simulink model "HVDC_VSC_1CPUcore_dcpl"  (Simulink 8.4)
settings: Solver=ode3  SolverMode=SingleTasking  StartTime=0.0  StopTime=70.0  FixedStep=Ts_Power  RelTol=1e-3  AbsTol=1e-2
PreLoadFcn:
  | Ts_Power=50e-6; Ts_Control=1*Ts_Power; init_cosim_IA; startup_transients_hvdc_vsc;
PostLoadFcn:
  | Ts_Power=50e-6; Ts_Control=1*Ts_Power; init_cosim_IA; startup_transients_hvdc_vsc;
InitFcn:
  | Ts_Power=50e-6; Ts_Control=1*Ts_Power; init_cosim_IA; startup_transients_hvdc_vsc;
undefined symbols (not defined in the file): CLARK, D1, Delta, dPref1_2, dPref1_2_rlimit, gcbh, h, intfDelay, level, lib_mesures, magnitude, ResistanceM, rte_drive_private_lib, rte_tsb3level_hiz_rect_cb, sps_rtmsupport, t_deblock_Pref1, t_deblock_Udref2, t_dPref1_2, t_SwitchITMIdc, t_SwitchITMVdc, Ts_intf, TSB3_hiZR
libraries: powerlib x183, spsVIMeasurementModel x102, powerlib_extras x71, powerlib_meascontrol x50, rteventslib x26, op_dpl_lib x20, rtlab x14, sps_avr x6, artemis x1
(part 8 of 13)

== system HVDC_VSC_1CPUcore_dcpl/SS_HVDCStation2_WSCC2/WSCC System 2/Bus_4 230 KV ==
  Three-Phase V-I Measurement1 : Subsystem  DialogController=POWERSYS.PowerSysDialog  LoadFcn=sps_rtmsupport('LoadFcn',gcbh);  StartFcn=sps_rtmsupport('StartFcn',gcbh);  StopFcn=sps_rtmsupport('StopFcn',gcbh);  mask(Three-Phase VI Measurement){VoltageMeasurement=phase-to-phase, SetLabelV=on, LabelV=Vabc_245, Vpu=off, VpuLL=off, CurrentMeasurement=yes, SetLabelI=on, LabelI=Iabc_245, Ipu=off, Pbase=100e6, Vbase=230e3, OutputType=Complex, PhasorSimulation=off, PSBequivalent=0}
      mask prompts: VoltageMeasurement "Voltage measurement"; SetLabelV "Use a label"; LabelV "Signal label  (use a From block to collect this signal)"; Vpu "Voltages in pu,  based on peak value of nominal phase-to-ground voltage"; VpuLL "Voltages in pu,  based on peak value of nominal phase-to-phase  voltage"; CurrentMeasurement "Current measurement"; SetLabelI "Use a label"; LabelI "Signal label  (use a From block to collect this signal)"; Ipu "Currents in pu"; Pbase "Base power ( VA 3 phase)"; Vbase "Nominal voltage used for pu measurement (Vrms phase-phase) :"; OutputType "Output signals in:"; PhasorSimulation "Phasor simulation (internal use)"; PSBequivalent "Equivalent circuit (internal use)"
      mask help:
      | Ideal three-phase voltage and current measurements.
      |
      | The block can output the voltages and currents in per unit values or in volts and amperes.
      mask init: same as HVDC_VSC_1CPUcore_dcpl/SM_WSCC1_HVDCStation1/B1
      settings: CopyFcn=sps_rtmsupport('CopyFcn',gcbh); powericon('ThreePhaseVIMeasurementCopy',gcb)  DeleteFcn=sps_rtmsupport('DeleteFcn',gcbh);  UndoDeleteFcn=sps_rtmsupport('UndoDeleteFcn',gcbh);  ModelCloseFcn=sps_rtmsupport('ModelCloseFcn',gcbh);  PreSaveFcn="sps_rtmsupport('PreSaveFcn',gcbh);  set_param(gcb,'LinkStatus','restore')"  PostSaveFcn=sps_rtmsupport('PostSaveFcn',gcbh);  NameChangeFcn=sps_rtmsupport('NameChangeFcn',gcbh);  PreCopyFcn=sps_rtmsupport('PreCopyFcn',gcbh);  OpenFcn=sps_rtmsupport('OpenFcn',gcbh, [1 2 4 5 6 7 9 -12 13]);  CloseFcn=sps_rtmsupport('CloseFcn',gcbh);  PreDeleteFcn=sps_rtmsupport('PreDeleteFcn',gcbh);
      mask Help: helpview(psbhelp)
      mask TypeOptions VoltageMeasurement: no | phase-to-ground | phase-to-phase
      mask Callback VoltageMeasurement: powericon('ThreePhaseVIMeasurementCback',gcb,'Vselector');
      mask Callback SetLabelV: powericon('ThreePhaseVIMeasurementCback',gcb,'');
      mask Callback Vpu: powericon('ThreePhaseVIMeasurementCback',gcb,'Vpu');
      mask Callback VpuLL: powericon('ThreePhaseVIMeasurementCback',gcb,'VpuLL');
      mask TypeOptions CurrentMeasurement: no | yes
      mask Callback CurrentMeasurement: powericon('ThreePhaseVIMeasurementCback',gcb,'');
      mask Callback SetLabelI: powericon('ThreePhaseVIMeasurementCback',gcb,'');
      mask Callback LabelI: powericon('ThreePhaseVIMeasurementCback',gcb,'');
      mask Callback Ipu: powericon('ThreePhaseVIMeasurementCback',gcb,'');
      mask TypeOptions OutputType: Complex | Real-Imag | Magnitude-Angle | Magnitude
  Three-Phase V-I Measurement3 : Subsystem  DialogController=POWERSYS.PowerSysDialog  LoadFcn=sps_rtmsupport('LoadFcn',gcbh);  StartFcn=sps_rtmsupport('StartFcn',gcbh);  StopFcn=sps_rtmsupport('StopFcn',gcbh);  mask(Three-Phase VI Measurement){VoltageMeasurement=phase-to-phase, SetLabelV=on, LabelV=Vabc_246, Vpu=off, VpuLL=off, CurrentMeasurement=yes, SetLabelI=on, LabelI=Iabc_246, Ipu=off, Pbase=100e6, Vbase=230e3, OutputType=Complex, PhasorSimulation=off, PSBequivalent=0}
      mask prompts: VoltageMeasurement "Voltage measurement"; SetLabelV "Use a label"; LabelV "Signal label  (use a From block to collect this signal)"; Vpu "Voltages in pu,  based on peak value of nominal phase-to-ground voltage"; VpuLL "Voltages in pu,  based on peak value of nominal phase-to-phase  voltage"; CurrentMeasurement "Current measurement"; SetLabelI "Use a label"; LabelI "Signal label  (use a From block to collect this signal)"; Ipu "Currents in pu"; Pbase "Base power ( VA 3 phase)"; Vbase "Nominal voltage used for pu measurement (Vrms phase-phase) :"; OutputType "Output signals in:"; PhasorSimulation "Phasor simulation (internal use)"; PSBequivalent "Equivalent circuit (internal use)"
      mask help:
      | Ideal three-phase voltage and current measurements.
      |
      | The block can output the voltages and currents in per unit values or in volts and amperes.
      mask init: same as HVDC_VSC_1CPUcore_dcpl/SM_WSCC1_HVDCStation1/B1
      settings: CopyFcn=sps_rtmsupport('CopyFcn',gcbh); powericon('ThreePhaseVIMeasurementCopy',gcb)  DeleteFcn=sps_rtmsupport('DeleteFcn',gcbh);  UndoDeleteFcn=sps_rtmsupport('UndoDeleteFcn',gcbh);  ModelCloseFcn=sps_rtmsupport('ModelCloseFcn',gcbh);  PreSaveFcn="sps_rtmsupport('PreSaveFcn',gcbh);  set_param(gcb,'LinkStatus','restore')"  PostSaveFcn=sps_rtmsupport('PostSaveFcn',gcbh);  NameChangeFcn=sps_rtmsupport('NameChangeFcn',gcbh);  PreCopyFcn=sps_rtmsupport('PreCopyFcn',gcbh);  OpenFcn=sps_rtmsupport('OpenFcn',gcbh, [1 2 4 5 6 7 9 -12 13]);  CloseFcn=sps_rtmsupport('CloseFcn',gcbh);  PreDeleteFcn=sps_rtmsupport('PreDeleteFcn',gcbh);
      mask Help: helpview(psbhelp)
      mask TypeOptions VoltageMeasurement: no | phase-to-ground | phase-to-phase
      mask Callback VoltageMeasurement: powericon('ThreePhaseVIMeasurementCback',gcb,'Vselector');
      mask Callback SetLabelV: powericon('ThreePhaseVIMeasurementCback',gcb,'');
      mask Callback Vpu: powericon('ThreePhaseVIMeasurementCback',gcb,'Vpu');
      mask Callback VpuLL: powericon('ThreePhaseVIMeasurementCback',gcb,'VpuLL');
      mask TypeOptions CurrentMeasurement: no | yes
      mask Callback CurrentMeasurement: powericon('ThreePhaseVIMeasurementCback',gcb,'');
      mask Callback SetLabelI: powericon('ThreePhaseVIMeasurementCback',gcb,'');
      mask Callback LabelI: powericon('ThreePhaseVIMeasurementCback',gcb,'');
      mask Callback Ipu: powericon('ThreePhaseVIMeasurementCback',gcb,'');
      mask TypeOptions OutputType: Complex | Real-Imag | Magnitude-Angle | Magnitude
  Conn7 : PMIOPort  Port=1  Side=Left
  Conn8 : PMIOPort  Port=2  Side=Left
  Conn9 : PMIOPort  Port=3  Side=Left
  Conn1 : PMIOPort  Port=4  Side=Right
  Conn2 : PMIOPort  Port=5  Side=Right
  Conn3 : PMIOPort  Port=6  Side=Right
  Conn4 : PMIOPort  Port=7  Side=Right
  Conn5 : PMIOPort  Port=8  Side=Right
  Conn6 : PMIOPort  Port=9  Side=Right
  connections:
  Three-Phase V-I Measurement3/LConn3 -- Conn9/RConn1 -- Three-Phase V-I Measurement1/LConn3
  Three-Phase V-I Measurement3/LConn2 -- Conn8/RConn1 -- Three-Phase V-I Measurement1/LConn2
  Three-Phase V-I Measurement3/LConn1 -- Conn7/RConn1 -- Three-Phase V-I Measurement1/LConn1
  Three-Phase V-I Measurement3/RConn3 -- Conn6/RConn1
  Three-Phase V-I Measurement1/RConn3 -- Conn3/RConn1
  Three-Phase V-I Measurement1/RConn1 -- Conn1/RConn1
  Three-Phase V-I Measurement1/RConn2 -- Conn2/RConn1
  Three-Phase V-I Measurement3/RConn1 -- Conn4/RConn1
  Three-Phase V-I Measurement3/RConn2 -- Conn5/RConn1

== system HVDC_VSC_1CPUcore_dcpl/SS_HVDCStation2_WSCC2/WSCC System 2/Bus_5 230 KV ==
  Kv : Gain  Gain=Ki  SaturateOnIntegerOverflow=on  OutDataTypeStr=Inherit: Same as input  ParamDataTypeStr=Inherit: Same as input
  Kv1 : Gain  Gain=Kv  SaturateOnIntegerOverflow=on  OutDataTypeStr=Inherit: Same as input  ParamDataTypeStr=Inherit: Same as input
  Mode I : spsVIMeasurementModel/Complex
  Mode V : spsVIMeasurementModel/Complex
  Model : spsVIMeasurementModel/VI_phase  SystemSampleTime=-1
  A : PMIOPort  Port=1  Side=Left
  B : PMIOPort  Port=2  Side=Left
  C : PMIOPort  Port=3  Side=Left
  a : PMIOPort  Port=4  Side=Right
  b : PMIOPort  Port=5  Side=Right
  c : PMIOPort  Port=6  Side=Right
  tag scope: Iabc_25=global, Vabc_25=global
  wires:
  Model/2 -> Kv/1
  Model/1 -> Kv1/1
  Kv/1 -> Mode I/1
  Kv1/1 -> Mode V/1
  Mode I/1 -> [Iabc_25]
  Mode V/1 -> [Vabc_25]
  connections:
  Model/RConn3 -- c/RConn1
  Model/RConn1 -- a/RConn1
  Model/RConn2 -- b/RConn1
  Model/LConn3 -- C/RConn1
  Model/LConn1 -- A/RConn1
  Model/LConn2 -- B/RConn1

== system HVDC_VSC_1CPUcore_dcpl/SS_HVDCStation2_WSCC2/WSCC System 2/Bus_6 230 KV ==
  Kv : Gain  Gain=Ki  SaturateOnIntegerOverflow=on  OutDataTypeStr=Inherit: Same as input  ParamDataTypeStr=Inherit: Same as input
  Kv1 : Gain  Gain=Kv  SaturateOnIntegerOverflow=on  OutDataTypeStr=Inherit: Same as input  ParamDataTypeStr=Inherit: Same as input
  Mode I : spsVIMeasurementModel/Complex
  Mode V : spsVIMeasurementModel/Complex
  Model : spsVIMeasurementModel/VI_phase  SystemSampleTime=-1
  A : PMIOPort  Port=1  Side=Left
  B : PMIOPort  Port=2  Side=Left
  C : PMIOPort  Port=3  Side=Left
  a : PMIOPort  Port=4  Side=Right
  b : PMIOPort  Port=5  Side=Right
  c : PMIOPort  Port=6  Side=Right
  tag scope: Iabc_26=global, Vabc_26=global
  wires:
  Model/2 -> Kv/1
  Model/1 -> Kv1/1
  Kv/1 -> Mode I/1
  Kv1/1 -> Mode V/1
  Mode I/1 -> [Iabc_26]
  Mode V/1 -> [Vabc_26]
  connections:
  Model/RConn3 -- c/RConn1
  Model/RConn1 -- a/RConn1
  Model/RConn2 -- b/RConn1
  Model/LConn3 -- C/RConn1
  Model/LConn1 -- A/RConn1
  Model/LConn2 -- B/RConn1

== system HVDC_VSC_1CPUcore_dcpl/SS_HVDCStation2_WSCC2/WSCC System 2/Bus_7 230 KV ==
  Three-Phase V-I Measurement1 : Subsystem  DialogController=POWERSYS.PowerSysDialog  LoadFcn=sps_rtmsupport('LoadFcn',gcbh);  StartFcn=sps_rtmsupport('StartFcn',gcbh);  StopFcn=sps_rtmsupport('StopFcn',gcbh);  mask(Three-Phase VI Measurement){VoltageMeasurement=phase-to-phase, SetLabelV=on, LabelV=Vabc_27, Vpu=off, VpuLL=off, CurrentMeasurement=yes, SetLabelI=on, LabelI=Iabc_27, Ipu=off, Pbase=100e6, Vbase=230e3, OutputType=Complex, PhasorSimulation=off, PSBequivalent=0}
      mask prompts: VoltageMeasurement "Voltage measurement"; SetLabelV "Use a label"; LabelV "Signal label  (use a From block to collect this signal)"; Vpu "Voltages in pu,  based on peak value of nominal phase-to-ground voltage"; VpuLL "Voltages in pu,  based on peak value of nominal phase-to-phase  voltage"; CurrentMeasurement "Current measurement"; SetLabelI "Use a label"; LabelI "Signal label  (use a From block to collect this signal)"; Ipu "Currents in pu"; Pbase "Base power ( VA 3 phase)"; Vbase "Nominal voltage used for pu measurement (Vrms phase-phase) :"; OutputType "Output signals in:"; PhasorSimulation "Phasor simulation (internal use)"; PSBequivalent "Equivalent circuit (internal use)"
      mask help:
      | Ideal three-phase voltage and current measurements.
      |
      | The block can output the voltages and currents in per unit values or in volts and amperes.
      mask init: same as HVDC_VSC_1CPUcore_dcpl/SM_WSCC1_HVDCStation1/B1
      settings: CopyFcn=sps_rtmsupport('CopyFcn',gcbh); powericon('ThreePhaseVIMeasurementCopy',gcb)  DeleteFcn=sps_rtmsupport('DeleteFcn',gcbh);  UndoDeleteFcn=sps_rtmsupport('UndoDeleteFcn',gcbh);  ModelCloseFcn=sps_rtmsupport('ModelCloseFcn',gcbh);  PreSaveFcn="sps_rtmsupport('PreSaveFcn',gcbh);  set_param(gcb,'LinkStatus','restore')"  PostSaveFcn=sps_rtmsupport('PostSaveFcn',gcbh);  NameChangeFcn=sps_rtmsupport('NameChangeFcn',gcbh);  PreCopyFcn=sps_rtmsupport('PreCopyFcn',gcbh);  OpenFcn=sps_rtmsupport('OpenFcn',gcbh, [1 2 4 5 6 7 9 -12 13]);  CloseFcn=sps_rtmsupport('CloseFcn',gcbh);  PreDeleteFcn=sps_rtmsupport('PreDeleteFcn',gcbh);
      mask Help: helpview(psbhelp)
      mask TypeOptions VoltageMeasurement: no | phase-to-ground | phase-to-phase
      mask Callback VoltageMeasurement: powericon('ThreePhaseVIMeasurementCback',gcb,'Vselector');
      mask Callback SetLabelV: powericon('ThreePhaseVIMeasurementCback',gcb,'');
      mask Callback Vpu: powericon('ThreePhaseVIMeasurementCback',gcb,'Vpu');
      mask Callback VpuLL: powericon('ThreePhaseVIMeasurementCback',gcb,'VpuLL');
      mask TypeOptions CurrentMeasurement: no | yes
      mask Callback CurrentMeasurement: powericon('ThreePhaseVIMeasurementCback',gcb,'');
      mask Callback SetLabelI: powericon('ThreePhaseVIMeasurementCback',gcb,'');
      mask Callback LabelI: powericon('ThreePhaseVIMeasurementCback',gcb,'');
      mask Callback Ipu: powericon('ThreePhaseVIMeasurementCback',gcb,'');
      mask TypeOptions OutputType: Complex | Real-Imag | Magnitude-Angle | Magnitude
  Three-Phase V-I Measurement3 : Subsystem  DialogController=POWERSYS.PowerSysDialog  LoadFcn=sps_rtmsupport('LoadFcn',gcbh);  StartFcn=sps_rtmsupport('StartFcn',gcbh);  StopFcn=sps_rtmsupport('StopFcn',gcbh);  mask(Three-Phase VI Measurement){VoltageMeasurement=phase-to-phase, SetLabelV=on, LabelV=Vabc_20, Vpu=off, VpuLL=off, CurrentMeasurement=yes, SetLabelI=on, LabelI=Iab_20, Ipu=off, Pbase=100e6, Vbase=230e3, OutputType=Complex, PhasorSimulation=off, PSBequivalent=0}
      mask prompts: VoltageMeasurement "Voltage measurement"; SetLabelV "Use a label"; LabelV "Signal label  (use a From block to collect this signal)"; Vpu "Voltages in pu,  based on peak value of nominal phase-to-ground voltage"; VpuLL "Voltages in pu,  based on peak value of nominal phase-to-phase  voltage"; CurrentMeasurement "Current measurement"; SetLabelI "Use a label"; LabelI "Signal label  (use a From block to collect this signal)"; Ipu "Currents in pu"; Pbase "Base power ( VA 3 phase)"; Vbase "Nominal voltage used for pu measurement (Vrms phase-phase) :"; OutputType "Output signals in:"; PhasorSimulation "Phasor simulation (internal use)"; PSBequivalent "Equivalent circuit (internal use)"
      mask help:
      | Ideal three-phase voltage and current measurements.
      |
      | The block can output the voltages and currents in per unit values or in volts and amperes.
      mask init: same as HVDC_VSC_1CPUcore_dcpl/SM_WSCC1_HVDCStation1/B1
      settings: CopyFcn=sps_rtmsupport('CopyFcn',gcbh); powericon('ThreePhaseVIMeasurementCopy',gcb)  DeleteFcn=sps_rtmsupport('DeleteFcn',gcbh);  UndoDeleteFcn=sps_rtmsupport('UndoDeleteFcn',gcbh);  ModelCloseFcn=sps_rtmsupport('ModelCloseFcn',gcbh);  PreSaveFcn="sps_rtmsupport('PreSaveFcn',gcbh);  set_param(gcb,'LinkStatus','restore')"  PostSaveFcn=sps_rtmsupport('PostSaveFcn',gcbh);  NameChangeFcn=sps_rtmsupport('NameChangeFcn',gcbh);  PreCopyFcn=sps_rtmsupport('PreCopyFcn',gcbh);  OpenFcn=sps_rtmsupport('OpenFcn',gcbh, [1 2 4 5 6 7 9 -12 13]);  CloseFcn=sps_rtmsupport('CloseFcn',gcbh);  PreDeleteFcn=sps_rtmsupport('PreDeleteFcn',gcbh);
      mask Help: helpview(psbhelp)
      mask TypeOptions VoltageMeasurement: no | phase-to-ground | phase-to-phase
      mask Callback VoltageMeasurement: powericon('ThreePhaseVIMeasurementCback',gcb,'Vselector');
      mask Callback SetLabelV: powericon('ThreePhaseVIMeasurementCback',gcb,'');
      mask Callback Vpu: powericon('ThreePhaseVIMeasurementCback',gcb,'Vpu');
      mask Callback VpuLL: powericon('ThreePhaseVIMeasurementCback',gcb,'VpuLL');
      mask TypeOptions CurrentMeasurement: no | yes
      mask Callback CurrentMeasurement: powericon('ThreePhaseVIMeasurementCback',gcb,'');
      mask Callback SetLabelI: powericon('ThreePhaseVIMeasurementCback',gcb,'');
      mask Callback LabelI: powericon('ThreePhaseVIMeasurementCback',gcb,'');
      mask Callback Ipu: powericon('ThreePhaseVIMeasurementCback',gcb,'');
      mask TypeOptions OutputType: Complex | Real-Imag | Magnitude-Angle | Magnitude
  Conn7 : PMIOPort  Port=1  Side=Left
  Conn8 : PMIOPort  Port=2  Side=Left
  Conn9 : PMIOPort  Port=3  Side=Left
  Conn1 : PMIOPort  Port=4  Side=Right
  Conn2 : PMIOPort  Port=5  Side=Right
  Conn3 : PMIOPort  Port=6  Side=Right
  Conn4 : PMIOPort  Port=7  Side=Right
  Conn5 : PMIOPort  Port=8  Side=Right
  Conn6 : PMIOPort  Port=9  Side=Right
  connections:
  Three-Phase V-I Measurement3/RConn2 -- Conn5/RConn1
  Three-Phase V-I Measurement3/RConn1 -- Conn4/RConn1
  Three-Phase V-I Measurement1/RConn2 -- Conn2/RConn1
  Three-Phase V-I Measurement1/RConn1 -- Conn1/RConn1
  Three-Phase V-I Measurement1/RConn3 -- Conn3/RConn1
  Three-Phase V-I Measurement3/RConn3 -- Conn6/RConn1
  Conn7/RConn1 -- Three-Phase V-I Measurement3/LConn3 -- Three-Phase V-I Measurement1/LConn1
  Conn8/RConn1 -- Three-Phase V-I Measurement3/LConn2 -- Three-Phase V-I Measurement1/LConn2
  Conn9/RConn1 -- Three-Phase V-I Measurement3/LConn1 -- Three-Phase V-I Measurement1/LConn3

== system HVDC_VSC_1CPUcore_dcpl/SS_HVDCStation2_WSCC2/WSCC System 2/Bus_8 230 KV ==
  Kv : Gain  Gain=Ki  SaturateOnIntegerOverflow=on  OutDataTypeStr=Inherit: Same as input  ParamDataTypeStr=Inherit: Same as input
  Kv1 : Gain  Gain=Kv  SaturateOnIntegerOverflow=on  OutDataTypeStr=Inherit: Same as input  ParamDataTypeStr=Inherit: Same as input
  Mode I : spsVIMeasurementModel/Complex
  Mode V : spsVIMeasurementModel/Complex
  Model : spsVIMeasurementModel/VI_phase  SystemSampleTime=-1
  A : PMIOPort  Port=1  Side=Left
  B : PMIOPort  Port=2  Side=Left
  C : PMIOPort  Port=3  Side=Left
  a : PMIOPort  Port=4  Side=Right
  b : PMIOPort  Port=5  Side=Right
  c : PMIOPort  Port=6  Side=Right
  tag scope: Iabc_28=global, Vabc_28=global
  wires:
  Model/2 -> Kv/1
  Model/1 -> Kv1/1
  Kv/1 -> Mode I/1
  Kv1/1 -> Mode V/1
  Mode I/1 -> [Iabc_28]
  Mode V/1 -> [Vabc_28]
  connections:
  Model/RConn3 -- c/RConn1
  Model/RConn1 -- a/RConn1
  Model/RConn2 -- b/RConn1
  Model/LConn3 -- C/RConn1
  Model/LConn1 -- A/RConn1
  Model/LConn2 -- B/RConn1

== system HVDC_VSC_1CPUcore_dcpl/SS_HVDCStation2_WSCC2/WSCC System 2/Bus_9 230 KV ==
  Three-Phase V-I Measurement1 : Subsystem  DialogController=POWERSYS.PowerSysDialog  LoadFcn=sps_rtmsupport('LoadFcn',gcbh);  StartFcn=sps_rtmsupport('StartFcn',gcbh);  StopFcn=sps_rtmsupport('StopFcn',gcbh);  mask(Three-Phase VI Measurement){VoltageMeasurement=phase-to-phase, SetLabelV=on, LabelV=Vabc_29, Vpu=off, VpuLL=off, CurrentMeasurement=yes, SetLabelI=on, LabelI=Iabc_29, Ipu=off, Pbase=100e6, Vbase=230e3, OutputType=Complex, PhasorSimulation=off, PSBequivalent=0}
      mask prompts: VoltageMeasurement "Voltage measurement"; SetLabelV "Use a label"; LabelV "Signal label  (use a From block to collect this signal)"; Vpu "Voltages in pu,  based on peak value of nominal phase-to-ground voltage"; VpuLL "Voltages in pu,  based on peak value of nominal phase-to-phase  voltage"; CurrentMeasurement "Current measurement"; SetLabelI "Use a label"; LabelI "Signal label  (use a From block to collect this signal)"; Ipu "Currents in pu"; Pbase "Base power ( VA 3 phase)"; Vbase "Nominal voltage used for pu measurement (Vrms phase-phase) :"; OutputType "Output signals in:"; PhasorSimulation "Phasor simulation (internal use)"; PSBequivalent "Equivalent circuit (internal use)"
      mask help:
      | Ideal three-phase voltage and current measurements.
      |
      | The block can output the voltages and currents in per unit values or in volts and amperes.
      mask init: same as HVDC_VSC_1CPUcore_dcpl/SM_WSCC1_HVDCStation1/B1
      settings: CopyFcn=sps_rtmsupport('CopyFcn',gcbh); powericon('ThreePhaseVIMeasurementCopy',gcb)  DeleteFcn=sps_rtmsupport('DeleteFcn',gcbh);  UndoDeleteFcn=sps_rtmsupport('UndoDeleteFcn',gcbh);  ModelCloseFcn=sps_rtmsupport('ModelCloseFcn',gcbh);  PreSaveFcn="sps_rtmsupport('PreSaveFcn',gcbh);  set_param(gcb,'LinkStatus','restore')"  PostSaveFcn=sps_rtmsupport('PostSaveFcn',gcbh);  NameChangeFcn=sps_rtmsupport('NameChangeFcn',gcbh);  PreCopyFcn=sps_rtmsupport('PreCopyFcn',gcbh);  OpenFcn=sps_rtmsupport('OpenFcn',gcbh, [1 2 4 5 6 7 9 -12 13]);  CloseFcn=sps_rtmsupport('CloseFcn',gcbh);  PreDeleteFcn=sps_rtmsupport('PreDeleteFcn',gcbh);
      mask Help: helpview(psbhelp)
      mask TypeOptions VoltageMeasurement: no | phase-to-ground | phase-to-phase
      mask Callback VoltageMeasurement: powericon('ThreePhaseVIMeasurementCback',gcb,'Vselector');
      mask Callback SetLabelV: powericon('ThreePhaseVIMeasurementCback',gcb,'');
      mask Callback Vpu: powericon('ThreePhaseVIMeasurementCback',gcb,'Vpu');
      mask Callback VpuLL: powericon('ThreePhaseVIMeasurementCback',gcb,'VpuLL');
      mask TypeOptions CurrentMeasurement: no | yes
      mask Callback CurrentMeasurement: powericon('ThreePhaseVIMeasurementCback',gcb,'');
      mask Callback SetLabelI: powericon('ThreePhaseVIMeasurementCback',gcb,'');
      mask Callback LabelI: powericon('ThreePhaseVIMeasurementCback',gcb,'');
      mask Callback Ipu: powericon('ThreePhaseVIMeasurementCback',gcb,'');
      mask TypeOptions OutputType: Complex | Real-Imag | Magnitude-Angle | Magnitude
  Three-Phase V-I Measurement3 : Subsystem  DialogController=POWERSYS.PowerSysDialog  LoadFcn=sps_rtmsupport('LoadFcn',gcbh);  StartFcn=sps_rtmsupport('StartFcn',gcbh);  StopFcn=sps_rtmsupport('StopFcn',gcbh);  mask(Three-Phase VI Measurement){VoltageMeasurement=phase-to-phase, SetLabelV=on, LabelV=Vabc_30, Vpu=off, VpuLL=off, CurrentMeasurement=yes, SetLabelI=on, LabelI=Iabc_30, Ipu=off, Pbase=100e6, Vbase=230e3, OutputType=Complex, PhasorSimulation=off, PSBequivalent=0}
      mask prompts: VoltageMeasurement "Voltage measurement"; SetLabelV "Use a label"; LabelV "Signal label  (use a From block to collect this signal)"; Vpu "Voltages in pu,  based on peak value of nominal phase-to-ground voltage"; VpuLL "Voltages in pu,  based on peak value of nominal phase-to-phase  voltage"; CurrentMeasurement "Current measurement"; SetLabelI "Use a label"; LabelI "Signal label  (use a From block to collect this signal)"; Ipu "Currents in pu"; Pbase "Base power ( VA 3 phase)"; Vbase "Nominal voltage used for pu measurement (Vrms phase-phase) :"; OutputType "Output signals in:"; PhasorSimulation "Phasor simulation (internal use)"; PSBequivalent "Equivalent circuit (internal use)"
      mask help:
      | Ideal three-phase voltage and current measurements.
      |
      | The block can output the voltages and currents in per unit values or in volts and amperes.
      mask init: same as HVDC_VSC_1CPUcore_dcpl/SM_WSCC1_HVDCStation1/B1
      settings: CopyFcn=sps_rtmsupport('CopyFcn',gcbh); powericon('ThreePhaseVIMeasurementCopy',gcb)  DeleteFcn=sps_rtmsupport('DeleteFcn',gcbh);  UndoDeleteFcn=sps_rtmsupport('UndoDeleteFcn',gcbh);  ModelCloseFcn=sps_rtmsupport('ModelCloseFcn',gcbh);  PreSaveFcn="sps_rtmsupport('PreSaveFcn',gcbh);  set_param(gcb,'LinkStatus','restore')"  PostSaveFcn=sps_rtmsupport('PostSaveFcn',gcbh);  NameChangeFcn=sps_rtmsupport('NameChangeFcn',gcbh);  PreCopyFcn=sps_rtmsupport('PreCopyFcn',gcbh);  OpenFcn=sps_rtmsupport('OpenFcn',gcbh, [1 2 4 5 6 7 9 -12 13]);  CloseFcn=sps_rtmsupport('CloseFcn',gcbh);  PreDeleteFcn=sps_rtmsupport('PreDeleteFcn',gcbh);
      mask Help: helpview(psbhelp)
      mask TypeOptions VoltageMeasurement: no | phase-to-ground | phase-to-phase
      mask Callback VoltageMeasurement: powericon('ThreePhaseVIMeasurementCback',gcb,'Vselector');
      mask Callback SetLabelV: powericon('ThreePhaseVIMeasurementCback',gcb,'');
      mask Callback Vpu: powericon('ThreePhaseVIMeasurementCback',gcb,'Vpu');
      mask Callback VpuLL: powericon('ThreePhaseVIMeasurementCback',gcb,'VpuLL');
      mask TypeOptions CurrentMeasurement: no | yes
      mask Callback CurrentMeasurement: powericon('ThreePhaseVIMeasurementCback',gcb,'');
      mask Callback SetLabelI: powericon('ThreePhaseVIMeasurementCback',gcb,'');
      mask Callback LabelI: powericon('ThreePhaseVIMeasurementCback',gcb,'');
      mask Callback Ipu: powericon('ThreePhaseVIMeasurementCback',gcb,'');
      mask TypeOptions OutputType: Complex | Real-Imag | Magnitude-Angle | Magnitude
  Conn7 : PMIOPort  Port=1  Side=Left
  Conn8 : PMIOPort  Port=2  Side=Left
  Conn9 : PMIOPort  Port=3  Side=Left
  Conn1 : PMIOPort  Port=4  Side=Right
  Conn2 : PMIOPort  Port=5  Side=Right
  Conn3 : PMIOPort  Port=6  Side=Right
  Conn10 : PMIOPort  Port=7  Side=Left
  Conn11 : PMIOPort  Port=8  Side=Left
  Conn12 : PMIOPort  Port=9  Side=Left
  connections:
  Conn9/RConn1 -- Three-Phase V-I Measurement1/LConn3
  Conn8/RConn1 -- Three-Phase V-I Measurement1/LConn2
  Conn7/RConn1 -- Three-Phase V-I Measurement1/LConn1
  Three-Phase V-I Measurement1/RConn3 -- Three-Phase V-I Measurement3/RConn3 -- Conn3/RConn1
  Three-Phase V-I Measurement1/RConn1 -- Three-Phase V-I Measurement3/RConn1 -- Conn1/RConn1
  Three-Phase V-I Measurement1/RConn2 -- Three-Phase V-I Measurement3/RConn2 -- Conn2/RConn1
  Conn10/RConn1 -- Three-Phase V-I Measurement3/LConn1
  Conn12/RConn1 -- Three-Phase V-I Measurement3/LConn3
  Conn11/RConn1 -- Three-Phase V-I Measurement3/LConn2

== system HVDC_VSC_1CPUcore_dcpl/SS_HVDCStation2_WSCC2/WSCC System 2/Generator BUS1x1 ==
  " Speed (pu)21" : Scope
      settings: TickLabels=on  TimeRange=100  YMin=0.995  YMax=1  SaveName=Gen21Freq
  247.5 MVA 16.5kV 3600 rpm2 : powerlib/Machines/Synchronous Machine pu Standard  PresetModel=No  MechanicalLoad=Mechanical power Pm  ShowDetailedParameters=on  RotorType=Round  Units=per unit standard parameters  MeasurementBus=off  NominalParameters="[ 247.5e6  16.5e3   60 ]"  Reactances1=[ 0.36135, 0.15048, 0.12375, 0.2475, 0.2398275, 0.12375, 0.08316 ]  Reactances2="[ 1.305, 0.296, 0.252, 0.474,  0.243,  0.18 ]"  dAxisTimeConstants=Open-circuit  qAxisTimeConstants=Open-circuit  TimeConstants1="[ 4.4849  0.0681  0.1  ]"  TimeConstants2="[ 8.96, 0.05,  0.31, 0.05 ]"  TimeConstants3="[  4.49  0.0681  0.0513  ]"  TimeConstants4=[ 8.0, 0.03, 0.3371, 0.0295 ]  TimeConstants5=[ 1.01, 0.053, 0.1 ]  TimeConstants6=[ 1.3201, 0.023, 1.0, 0.07 ]  TimeConstants7="[  1.01  0.053  0.051266  ]"  TimeConstants8=[ 1.3201, 0.0231, 0.3371, 0.0295 ]  StatorResistance=0.000125  Mechanical="[ 23.64  0 1 ]"  PolePairs=1  InitialConditions=[0 -86.3058 0.296671 0.296671 0.296671 -20.4087 -140.409 99.5913 1.08165]  SetSaturation=off  Saturation=[0.6404,0.7127,0.8441,0.9214,0.9956,1.082,1.19,1.316,1.457;0.7,0.7698,0.8872,0.9466,0.9969,1.046,1.1,1.151,1.201]  LoadFlowParameters=[2 71600000 0 0 0]  TsPowergui=0  TsBlock=-1  IterativeModel=Trapezoidal non iterative  BusType=swing  Pref=0  Qref=0  Qmin=-Inf  Qmax=Inf  PLF=0  QLF=0
  Bus Selector3 : BusSelector  OutputSignals="Output active power   Peo (pu),Output reactive power  Qeo (pu),dq0 components.Stator voltage  vd (pu),dq0 components.Stator voltage  vq (pu),Mechanical.Rotor angle deviation  d_theta (rad),Mechanical.Rotor speed  wm  (pu),Mechanical.Rotor speed deviation  dw (pu)"
  Constant1 : Constant
  Excitation System2 : sps_avr/Excitation System  tr=20e-3  reg=[ 200, 0.02 ]  exc=[ 1, 0 ]  tgr=[ 12.0, 1.0 ]  damp=[ 0.03, 1.0 ]  sat=[ 0, 0 ]  lim=[ -10.0, 10.0, 0 ]  v0=[1.04 1.0817]
  Gain : Gain  Gain=247.5e6
  Gain1 : Gain  Gain=247.5e6
  Ground2 : Ground
  Pref2 : Constant  Value=0.28917
  Steam Turbine and Governor1 : powerlib/Machines/Steam Turbine and Governor  gentype=Tandem-compound (single mass)  reg1="[ 1  0.05    0 ]"  reg2="[ 0.001  0.1 ]"  reg3="[ -10.0 0.1   0.1 1.0 ]"  N=3600  turb1="[ 0.12  0.13  10.0   0.32   ]"  turb2="[ 0.48   0.25   0  0.27 ]"  HA="[  1.5498   0.24894  0  0 ]"  KA="[  83.47  42.702  0  0 ]"  DA="[  0.3104  0.05  0  0 ]*8"  ini1=0.28918  ini2=[1.88924e-008,-120.067]
  Subsystem1 : Subsystem
  Terminator1 : Terminator
  Turbine21 : Scope  NumInputPorts=2
      settings: TimeRange=0.5  YMin=0~-1  YMax=3e+09~1  SaveName=ScopeData2
  Va Gen21 : Scope
      settings: TickLabels=on  TimeRange=2  YMin=-15000  YMax=15000  SaveName=vf4
  Va4 : powerlib/Measurements/Voltage Measurement  Tag=PoWeRsYsTeMmEaSuReMeNt  PhasorSimulation=off  OutputType=Magnitude  PSBequivalent=0
  Vref2 : Constant  Value=1.04
  output Ground5 : powerlib/Elements/Ground  LConnTagsString=a
  A : PMIOPort  Port=1  Side=Right
  B : PMIOPort  Port=2  Side=Right
  C : PMIOPort  Port=3  Side=Right
  tag scope: OmegaGen21=global, Pgen21=global, Qgen21=global
  wires:
  Constant1/1 -> Steam Turbine and Governor1/1
  Bus Selector3/5 -> Steam Turbine and Governor1/4  "<Rotor angle deviation  d_theta (rad)>"
  Subsystem1/2(T_23) -> Turbine21/2  "T2 (Gen-LP)  T3(LP-HP)  [pu]"
  Steam Turbine and Governor1/3 -> Terminator1/1
  Bus Selector3/7 -> Subsystem1/1(In1)  "<Rotor speed deviation  dw (pu)>"
  Vref2/1 -> Excitation System2/1
  Pref2/1 -> Steam Turbine and Governor1/2
  Steam Turbine and Governor1/1 -> Subsystem1/2(In2)
  Subsystem1/1(dw_123) -> Turbine21/1  "dw1(Gen)  dw2(LP)   dw3(HP) [pu]"
  Steam Turbine and Governor1/4 -> 247.5 MVA 16.5kV 3600 rpm2/1
  Steam Turbine and Governor1/2 -> Subsystem1/3(In3)
  Bus Selector3/6 -> [OmegaGen21], " Speed (pu)21"/1, Steam Turbine and Governor1/3  "<Rotor speed  wm  (pu)>"
  247.5 MVA 16.5kV 3600 rpm2/1 -> Bus Selector3/1
  Ground2/1 -> Excitation System2/4
  Bus Selector3/4 -> Excitation System2/3  "<Stator voltage  vq (pu)>"
  Bus Selector3/3 -> Excitation System2/2  "<Stator voltage  vd (pu)>"
  Excitation System2/1 -> 247.5 MVA 16.5kV 3600 rpm2/2
  Va4/1 -> Va Gen21/1
  Bus Selector3/1 -> Gain/1  "<Output active power   Peo (pu)>"
  Bus Selector3/2 -> Gain1/1  "<Output reactive power  Qeo (pu)>"
  Gain/1 -> [Pgen21]
  Gain1/1 -> [Qgen21]
  connections:
  output Ground5/LConn1 -- Va4/LConn2
  C/RConn1 -- 247.5 MVA 16.5kV 3600 rpm2/RConn3
  247.5 MVA 16.5kV 3600 rpm2/RConn2 -- B/RConn1
  Va4/LConn1 -- 247.5 MVA 16.5kV 3600 rpm2/RConn1 -- A/RConn1

== system HVDC_VSC_1CPUcore_dcpl/SS_HVDCStation2_WSCC2/WSCC System 2/Generator BUS2x1 ==
  " Speed (pu)22" : Scope
      settings: TickLabels=on  TimeRange=150  YMin=0.995  YMax=1  SaveName=Pm2
  192 MVA 18kV 3600 rpm2 : powerlib/Machines/Synchronous Machine pu Standard  PresetModel=No  MechanicalLoad=Mechanical power Pm  ShowDetailedParameters=on  RotorType=Round  Units=per unit standard parameters  MeasurementBus=off  NominalParameters="[ 192e6  18e3   60 ]"  Reactances1=[ 1.719936, 0.230016, 0.1632, 1.65984, 0.378048, 0.2304, 0.10002 ]  Reactances2="[ 1.305, 0.296, 0.252, 0.474,  0.243,  0.18 ]"  dAxisTimeConstants=Open-circuit  qAxisTimeConstants=Open-circuit  TimeConstants1="[ 4.4849  0.0681  0.1  ]"  TimeConstants2="[ 6.0, 0.05,  0.535, 0.05 ]"  TimeConstants3="[  4.49  0.0681  0.0513  ]"  TimeConstants4=[ 8.0, 0.03, 0.3371, 0.0295 ]  TimeConstants5=[ 1.01, 0.053, 0.1 ]  TimeConstants6=[ 1.3201, 0.023, 1.0, 0.07 ]  TimeConstants7="[  1.01  0.053  0.051266  ]"  TimeConstants8=[ 1.3201, 0.0231, 0.3371, 0.0295 ]  StatorResistance=0.000125  Mechanical="[ 6.4  0 1 ]"  PolePairs=1  InitialConditions=[0 -28.9349 0.828916 0.828916 0.828916 6.92884 -113.071 126.929 1.78871]  SetSaturation=off  Saturation=[0.6404,0.7127,0.8441,0.9214,0.9956,1.082,1.19,1.316,1.457;0.7,0.7698,0.8872,0.9466,0.9969,1.046,1.1,1.151,1.201]  LoadFlowParameters=[1 163000000 0 0 0]  TsPowergui=0  TsBlock=-1  IterativeModel=Trapezoidal non iterative  BusType=PV  Pref=163e6  Qref=0  Qmin=-Inf  Qmax=Inf  PLF=0  QLF=0
  Bus Selector3 : BusSelector  OutputSignals="Output active power   Peo (pu),Output reactive power  Qeo (pu),dq0 components.Stator voltage  vd (pu),dq0 components.Stator voltage  vq (pu),Mechanical.Rotor angle deviation  d_theta (rad),Mechanical.Rotor speed  wm  (pu),Mechanical.Rotor speed deviation  dw (pu)"
  Constant1 : Constant
  Excitation System2 : sps_avr/Excitation System  tr=20e-3  reg=[ 200, 0.02 ]  exc=[ 1, 0 ]  tgr=[ 12.0, 1.0 ]  damp=[ 0.03, 1.0 ]  sat=[ 0, 0 ]  lim=[ -10.0, 10.0, 0 ]  v0=[1.025 1.7887]
  Gain : Gain  Gain=192e6
  Gain1 : Gain  Gain=192e6
  Ground2 : Ground
  Pref2 : Constant  Value=0.84896
  Steam Turbine and Governor1 : powerlib/Machines/Steam Turbine and Governor  gentype=Tandem-compound (single mass)  reg1="[ 1  0.05    0 ]"  reg2="[ 0.001  0.1 ]"  reg3="[ -10.0 0.1   0.1 1.0 ]"  N=3600  turb1="[ 0.12  0.13  10.0   0.32   ]"  turb2="[ 0.48   0.25   0  0.27 ]"  HA="[  1.5498   0.24894  0  0 ]"  KA="[  83.47  42.702  0  0 ]"  DA="[  0.3104  0.05  0  0 ]*8"  ini1=0.84904  ini2=[1.88924e-008,-120.067]
  Subsystem1 : Subsystem
  Terminator1 : Terminator
  Turbine22 : Scope  NumInputPorts=2
      settings: TimeRange=0.5  YMin=-0.03~-5  YMax=0.03~5  SaveName=ScopeData2
  Va Gen22 : Scope
      settings: TickLabels=on  TimeRange=150  YMin=-20000  YMax=20000  SaveName=vf4
  Va4 : powerlib/Measurements/Voltage Measurement  Tag=PoWeRsYsTeMmEaSuReMeNt  PhasorSimulation=off  OutputType=Magnitude  PSBequivalent=0
  Vref2 : Constant  Value=1.025
  output Ground5 : powerlib/Elements/Ground  LConnTagsString=a
  A : PMIOPort  Port=1  Side=Right
  B : PMIOPort  Port=2  Side=Right
  C : PMIOPort  Port=3  Side=Right
  tag scope: OmegaGen22=global, Pgen22=global, Qgen22=global
  wires:
  Constant1/1 -> Steam Turbine and Governor1/1
  Bus Selector3/5 -> Steam Turbine and Governor1/4  "<Rotor angle deviation  d_theta (rad)>"
  Subsystem1/2(T_23) -> Turbine22/2  "T2 (Gen-LP)  T3(LP-HP)  [pu]"
  Steam Turbine and Governor1/3 -> Terminator1/1
  Bus Selector3/7 -> Subsystem1/1(In1)  "<Rotor speed deviation  dw (pu)>"
  Vref2/1 -> Excitation System2/1
  Pref2/1 -> Steam Turbine and Governor1/2
  Steam Turbine and Governor1/1 -> Subsystem1/2(In2)
  Subsystem1/1(dw_123) -> Turbine22/1  "dw1(Gen)  dw2(LP)   dw3(HP) [pu]"
  Steam Turbine and Governor1/4 -> 192 MVA 18kV 3600 rpm2/1
  Steam Turbine and Governor1/2 -> Subsystem1/3(In3)
  Bus Selector3/6 -> [OmegaGen22], " Speed (pu)22"/1, Steam Turbine and Governor1/3  "<Rotor speed  wm  (pu)>"
  192 MVA 18kV 3600 rpm2/1 -> Bus Selector3/1
  Ground2/1 -> Excitation System2/4
  Bus Selector3/4 -> Excitation System2/3  "<Stator voltage  vq (pu)>"
  Bus Selector3/3 -> Excitation System2/2  "<Stator voltage  vd (pu)>"
  Excitation System2/1 -> 192 MVA 18kV 3600 rpm2/2
  Va4/1 -> Va Gen22/1
  Bus Selector3/2 -> Gain1/1  "<Output reactive power  Qeo (pu)>"
  Bus Selector3/1 -> Gain/1  "<Output active power   Peo (pu)>"
  Gain/1 -> [Pgen22]
  Gain1/1 -> [Qgen22]
  connections:
  output Ground5/LConn1 -- Va4/LConn2
  C/RConn1 -- 192 MVA 18kV 3600 rpm2/RConn3
  192 MVA 18kV 3600 rpm2/RConn2 -- B/RConn1
  Va4/LConn1 -- 192 MVA 18kV 3600 rpm2/RConn1 -- A/RConn1

== system HVDC_VSC_1CPUcore_dcpl/SS_HVDCStation2_WSCC2/WSCC System 2/Generator BUS3x1 ==
  " Speed (pu)23" : Scope
      settings: TickLabels=on  TimeRange=150  YMin=0.99955  YMax=1  SaveName=Pm2
  128 MVA 13.8kV 3600 rpm2 : powerlib/Machines/Synchronous Machine pu Standard  PresetModel=No  MechanicalLoad=Mechanical power Pm  ShowDetailedParameters=on  RotorType=Round  Units=per unit standard parameters  MeasurementBus=off  NominalParameters="[ 128e6  13.8e3   60 ]"  Reactances1=[ 1.68, 0.232064, 0.1536, 1.609984, 0.32, 0.2176, 0.094976 ]  Reactances2="[ 1.305, 0.296, 0.252, 0.474,  0.243,  0.18 ]"  dAxisTimeConstants=Open-circuit  qAxisTimeConstants=Open-circuit  TimeConstants1="[ 4.4849  0.0681  0.1  ]"  TimeConstants2="[ 5.89, 0.05,  0.6, 0.05 ]"  TimeConstants3="[  4.49  0.0681  0.0513  ]"  TimeConstants4=[ 8.0, 0.03, 0.3371, 0.0295 ]  TimeConstants5=[ 1.01, 0.053, 0.1 ]  TimeConstants6=[ 1.3201, 0.023, 1.0, 0.07 ]  TimeConstants7="[  1.01  0.053  0.051266  ]"  TimeConstants8=[ 1.3201, 0.0231, 0.3371, 0.0295 ]  StatorResistance=0.000125  Mechanical="[ 3.01  0 1 ]"  PolePairs=1  InitialConditions=[0 -35.8791 0.653244 0.653244 0.653244 11.9635 -108.037 131.963 1.40212]  SetSaturation=off  Saturation=[0.6404,0.7127,0.8441,0.9214,0.9956,1.082,1.19,1.316,1.457;0.7,0.7698,0.8872,0.9466,0.9969,1.046,1.1,1.151,1.201]  LoadFlowParameters=[1 85000000 0 0 0]  TsPowergui=0  TsBlock=-1  IterativeModel=Trapezoidal non iterative  BusType=PV  Pref=85e6  Qref=0  Qmin=-Inf  Qmax=Inf  PLF=0  QLF=0
  Bus Selector3 : BusSelector  OutputSignals="Output active power   Peo (pu),Output reactive power  Qeo (pu),dq0 components.Stator voltage  vd (pu),dq0 components.Stator voltage  vq (pu),Mechanical.Rotor angle deviation  d_theta (rad),Mechanical.Rotor speed  wm  (pu),Mechanical.Rotor speed deviation  dw (pu)"
  Constant1 : Constant
  Excitation System2 : sps_avr/Excitation System  tr=20e-3  reg=[ 200, 0.02 ]  exc=[ 1, 0 ]  tgr=[ 12.0, 1.0 ]  damp=[ 0.03, 1.0 ]  sat=[ 0, 0 ]  lim=[ -10.0, 10.0, 0 ]  v0=[1.025 1.4021]
  Gain : Gain  Gain=128e6
  Gain1 : Gain  Gain=128e6
  Ground2 : Ground
  Pref2 : Constant  Value=0.66406
  Steam Turbine and Governor1 : powerlib/Machines/Steam Turbine and Governor  gentype=Tandem-compound (single mass)  reg1="[ 1  0.05    0 ]"  reg2="[ 0.001  0.1 ]"  reg3="[ -10.0 0.1   0.1 1.0 ]"  N=3600  turb1="[ 0.12  0.13  10.0   0.32   ]"  turb2="[ 0.48   0.25   0  0.27 ]"  HA="[  1.5498   0.24894  0  0 ]"  KA="[  83.47  42.702  0  0 ]"  DA="[  0.3104  0.05  0  0 ]*8"  ini1=0.66412  ini2=[1.88924e-008,-120.067]
  Subsystem1 : Subsystem
  Terminator1 : Terminator
  Turbine23 : Scope  NumInputPorts=2
      settings: TimeRange=0.5  YMin=-3e-07~-1  YMax=5e-08~1  SaveName=ScopeData2
  Va Gen23 : Scope
      settings: TickLabels=on  TimeRange=0.007300652369719236  YMin=-15000  YMax=15000  SaveName=vf4
  Va4 : powerlib/Measurements/Voltage Measurement  Tag=PoWeRsYsTeMmEaSuReMeNt  PhasorSimulation=off  OutputType=Magnitude  PSBequivalent=0
  Vref2 : Constant  Value=1.025
  output Ground5 : powerlib/Elements/Ground  LConnTagsString=a
  A : PMIOPort  Port=1  Side=Right
  B : PMIOPort  Port=2  Side=Right
  C : PMIOPort  Port=3  Side=Right
  tag scope: OmegaGen23=global, Pgen23=global, Qgen23=global
  wires:
  Constant1/1 -> Steam Turbine and Governor1/1
  Bus Selector3/5 -> Steam Turbine and Governor1/4  "<Rotor angle deviation  d_theta (rad)>"
  Subsystem1/2(T_23) -> Turbine23/2  "T2 (Gen-LP)  T3(LP-HP)  [pu]"
  Steam Turbine and Governor1/3 -> Terminator1/1
  Bus Selector3/7 -> Subsystem1/1(In1)  "<Rotor speed deviation  dw (pu)>"
  Vref2/1 -> Excitation System2/1
  Pref2/1 -> Steam Turbine and Governor1/2
  Steam Turbine and Governor1/1 -> Subsystem1/2(In2)
  Subsystem1/1(dw_123) -> Turbine23/1  "dw1(Gen)  dw2(LP)   dw3(HP) [pu]"
  Steam Turbine and Governor1/4 -> 128 MVA 13.8kV 3600 rpm2/1
  Steam Turbine and Governor1/2 -> Subsystem1/3(In3)
  Bus Selector3/6 -> [OmegaGen23], " Speed (pu)23"/1, Steam Turbine and Governor1/3  "<Rotor speed  wm  (pu)>"
  128 MVA 13.8kV 3600 rpm2/1 -> Bus Selector3/1
  Ground2/1 -> Excitation System2/4
  Bus Selector3/4 -> Excitation System2/3  "<Stator voltage  vq (pu)>"
  Bus Selector3/3 -> Excitation System2/2  "<Stator voltage  vd (pu)>"
  Excitation System2/1 -> 128 MVA 13.8kV 3600 rpm2/2
  Va4/1 -> Va Gen23/1
  Gain/1 -> [Pgen23]
  Bus Selector3/1 -> Gain/1  "<Output active power   Peo (pu)>"
  Gain1/1 -> [Qgen23]
  Bus Selector3/2 -> Gain1/1  "<Output reactive power  Qeo (pu)>"
  connections:
  output Ground5/LConn1 -- Va4/LConn2
  C/RConn1 -- 128 MVA 13.8kV 3600 rpm2/RConn3
  128 MVA 13.8kV 3600 rpm2/RConn2 -- B/RConn1
  Va4/LConn1 -- 128 MVA 13.8kV 3600 rpm2/RConn1 -- A/RConn1

== system HVDC_VSC_1CPUcore_dcpl/SS_HVDCStation2_WSCC2/WSCC System 2/Three-Phase V-I Measurement ==
  Kv : Gain  Gain=Ki  SaturateOnIntegerOverflow=on  OutDataTypeStr=Inherit: Same as input  ParamDataTypeStr=Inherit: Same as input
  Kv1 : Gain  Gain=Kv  SaturateOnIntegerOverflow=on  OutDataTypeStr=Inherit: Same as input  ParamDataTypeStr=Inherit: Same as input
  Mode I : spsVIMeasurementModel/Complex
  Mode V : spsVIMeasurementModel/Complex
  Model : spsVIMeasurementModel/VI  SystemSampleTime=-1
  A : PMIOPort  Port=1  Side=Left
  B : PMIOPort  Port=2  Side=Left
  C : PMIOPort  Port=3  Side=Left
  a : PMIOPort  Port=4  Side=Right
  b : PMIOPort  Port=5  Side=Right
  c : PMIOPort  Port=6  Side=Right
  Vabc : Outport
  Iabc : Outport  Port=2
  wires:
  Model/2 -> Kv/1
  Model/1 -> Kv1/1
  Kv/1 -> Mode I/1
  Kv1/1 -> Mode V/1
  Mode I/1 -> Iabc/1
  Mode V/1 -> Vabc/1
  connections:
  Model/RConn3 -- c/RConn1
  Model/RConn1 -- a/RConn1
  Model/RConn2 -- b/RConn1
  Model/LConn3 -- C/RConn1
  Model/LConn1 -- A/RConn1
  Model/LConn2 -- B/RConn1

== system HVDC_VSC_1CPUcore_dcpl/SS_HVDCStation2_WSCC2/WSCC System 2/Three-Phase V-I Measurement2 ==
  Kv : Gain  Gain=Ki  SaturateOnIntegerOverflow=on  OutDataTypeStr=Inherit: Same as input  ParamDataTypeStr=Inherit: Same as input
  Kv1 : Gain  Gain=Kv  SaturateOnIntegerOverflow=on  OutDataTypeStr=Inherit: Same as input  ParamDataTypeStr=Inherit: Same as input
  Mode I : spsVIMeasurementModel/Complex
  Mode V : spsVIMeasurementModel/Complex
  Model : spsVIMeasurementModel/VI  SystemSampleTime=-1
  A : PMIOPort  Port=1  Side=Left
  B : PMIOPort  Port=2  Side=Left
  C : PMIOPort  Port=3  Side=Left
  a : PMIOPort  Port=4  Side=Right
  b : PMIOPort  Port=5  Side=Right
  c : PMIOPort  Port=6  Side=Right
  Vabc : Outport
  Iabc : Outport  Port=2
  wires:
  Mode V/1 -> Vabc/1
  Mode I/1 -> Iabc/1
  Kv1/1 -> Mode V/1
  Kv/1 -> Mode I/1
  Model/1 -> Kv1/1
  Model/2 -> Kv/1
  connections:
  Model/LConn2 -- B/RConn1
  Model/LConn1 -- A/RConn1
  Model/LConn3 -- C/RConn1
  Model/RConn2 -- b/RConn1
  Model/RConn1 -- a/RConn1
  Model/RConn3 -- c/RConn1

== system HVDC_VSC_1CPUcore_dcpl/SM_WSCC1_HVDCStation1/Station 1 (Rectifier)/TSB3_hiZR2/Subsystem ==
  I+ : Inport
  I- : Inport  Port=2
  In : Inport  Port=3
  common : Inport  Port=4
  enable : Inport  Port=5
  Add : Sum  Inputs=+
  Add1 : Sum  Inputs=+-
  Demux2 : Demux  Outputs=3
  Mux3 : Mux  Inputs=3
  Product : Product  SaturateOnIntegerOverflow=on  InputSameDT=on  OutDataTypeStr=Inherit: Same as first input
  Switch : Switch  Threshold=0.5
  common mode removal : Gain  Gain=1/3  SaturateOnIntegerOverflow=on  OutDataTypeStr=Inherit: Same as input  ParamDataTypeStr=Inherit: Same as input
  I+. : Outport
  I-. : Outport  Port=2
  In. : Outport  Port=3
  wires:
  Mux3/1 -> Add/1, Switch/3, Add1/1
  Add/1 -> common mode removal/1
  I+/1 -> Mux3/1
  I-/1 -> Mux3/2
  In/1 -> Mux3/3
  Demux2/1 -> I+./1
  Demux2/2 -> I-./1
  Demux2/3 -> In./1
  common/1 -> Switch/2
  Add1/1 -> Switch/1
  common mode removal/1 -> Add1/2
  Switch/1 -> Product/1
  Product/1 -> Demux2/1
  enable/1 -> Product/2

== system HVDC_VSC_1CPUcore_dcpl/SM_WSCC1_HVDCStation1/Station 1 (Rectifier)/TSB3_hiZR2/breaker model ==
  note: Current Prediction
  note: Zero crossing detection
  v : Inport
  g : Inport  Port=2
  0 1 : Constant  Value=0
  >1.5 : Relay  OnSwitchValue=1.5  OffSwitchValue=0
  Data Type  Conversion : DataTypeConversion  OutDataTypeStr=double  SaturateOnIntegerOverflow=on  RndMeth=Zero
  Data Type  Conversion1 : DataTypeConversion  OutDataTypeStr=boolean  SaturateOnIntegerOverflow=on  RndMeth=Zero
  Data Type  Conversion2 : DataTypeConversion  OutDataTypeStr=double  SaturateOnIntegerOverflow=on  RndMeth=Zero
  Data Type  Conversion3 : DataTypeConversion  OutDataTypeStr=boolean  SaturateOnIntegerOverflow=on  RndMeth=Zero
  Data Type  Conversion4 : DataTypeConversion  OutDataTypeStr=double  SaturateOnIntegerOverflow=on  RndMeth=Zero
  Gain : Gain  Gain=2  SaturateOnIntegerOverflow=on  OutDataTypeStr=Inherit: Same as input  ParamDataTypeStr=Inherit: Same as input
  IC : InitialCondition  Value=[0 0 0]
  Mem1 : Memory  InheritSampleTime=on
  Mem9 : Memory  InheritSampleTime=on
  Product : Product  SaturateOnIntegerOverflow=on  InputSameDT=on  OutDataTypeStr=Inherit: Same as first input
  Sum : Sum  Inputs=+-  SaturateOnIntegerOverflow=on  InputSameDT=on  OutDataTypeStr=Inherit: Same as first input
  b5 : RelationalOperator  Operator=>  InputSameDT=on
  or : Logic  Operator=OR
  sum : Sum  SaturateOnIntegerOverflow=on  InputSameDT=on  OutDataTypeStr=Inherit: Same as first input
  Status : Outport  InitialOutput=0
  wires:
  Gain/1 -> Sum/1
  Mem9/1 -> Sum/2
  v/1 -> Gain/1, Mem9/1  "Braeker voltage"
  Sum/1 -> Product/1, Mem1/1
  Mem1/1 -> Product/2
  0 1/1 -> b5/2
  Data Type  Conversion2/1 -> sum/1
  sum/1 -> >1.5/1
  g/1 -> Data Type  Conversion3/1, Data Type  Conversion4/1
  >1.5/1 -> Data Type  Conversion1/1
  Data Type  Conversion3/1 -> or/2
  Data Type  Conversion1/1 -> or/1
  IC/1 -> Status/1
  or/1 -> Data Type  Conversion/1
  Data Type  Conversion/1 -> IC/1
  b5/1 -> Data Type  Conversion2/1
  Product/1 -> b5/1
  Data Type  Conversion4/1 -> sum/2

== system HVDC_VSC_1CPUcore_dcpl/SM_WSCC1_HVDCStation1/VSC Controller (Station 1)/3-level firing pulse unit for TSB/Carriers Generator ==
  theta : Inport
  Constant2 : Constant  Value=0.5
  Gain1 : Gain  Gain=1/pi  SaturateOnIntegerOverflow=on  OutDataTypeStr=Inherit: Same as input  ParamDataTypeStr=Inherit: Same as input
  Sum1 : Sum  SaturateOnIntegerOverflow=on  InputSameDT=on  OutDataTypeStr=Inherit: Same as first input
  Sum2 : Sum  Inputs=+-  SaturateOnIntegerOverflow=on  InputSameDT=on  OutDataTypeStr=Inherit: Same as first input
  Trigonometric Function : Trigonometry  Operator=asin
  Trigonometric Function3 : Trigonometry
  C+ : Outport
  C- : Outport  Port=2
  wires:
  Trigonometric Function/1 -> Gain1/1
  Trigonometric Function3/1 -> Trigonometric Function/1
  Gain1/1 -> Sum1/1, Sum2/1
  Constant2/1 -> Sum2/2, Sum1/2
  Sum2/1 -> C-/1  "Carrier 1-"
  Sum1/1 -> C+/1  "Carrier 1+"
  theta/1 -> Trigonometric Function3/1

== system HVDC_VSC_1CPUcore_dcpl/SM_WSCC1_HVDCStation1/VSC Controller (Station 1)/3-level firing pulse unit for TSB/Subsystem1 ==
  in : Inport
  c+ : Inport  Port=2
  c- : Inport  Port=3
  RTE Logical Operator : rteventslib/Math Operations/RTE Logical Operator  LogicalOperator=NOT  NbrInput=1  NbrMaxEvents=1
  RTE Logical Operator1 : rteventslib/Math Operations/RTE Logical Operator  LogicalOperator=NOT  NbrInput=1  NbrMaxEvents=1
  RTE Relational Operator2 : rteventslib/Math Operations/RTE Relational Operator  RelationalOperator=>=  NumberMaxEvents=1  SampleTime=Ts
  RTE Relational Operator3 : rteventslib/Math Operations/RTE Relational Operator  RelationalOperator=<=  NumberMaxEvents=1  SampleTime=Ts
  1 : Outport
  2 : Outport  Port=2
  3 : Outport  Port=3
  4 : Outport  Port=4
  wires:
  in/1 -> RTE Relational Operator3/1, RTE Relational Operator2/1
  c+/1 -> RTE Relational Operator2/2
  c-/1 -> RTE Relational Operator3/2
  RTE Relational Operator2/1 -> RTE Logical Operator/1, 1/1
  RTE Relational Operator3/1 -> RTE Logical Operator1/1, 4/1
  RTE Logical Operator1/1 -> 2/1
  RTE Logical Operator/1 -> 3/1

== system HVDC_VSC_1CPUcore_dcpl/SM_WSCC1_HVDCStation1/VSC Controller (Station 1)/3-level firing pulse unit for TSB/Subsystem2 ==
  in : Inport
  c+ : Inport  Port=2
  c- : Inport  Port=3
  RTE Logical Operator : rteventslib/Math Operations/RTE Logical Operator  LogicalOperator=NOT  NbrInput=1  NbrMaxEvents=1
  RTE Logical Operator1 : rteventslib/Math Operations/RTE Logical Operator  LogicalOperator=NOT  NbrInput=1  NbrMaxEvents=1
  RTE Relational Operator2 : rteventslib/Math Operations/RTE Relational Operator  RelationalOperator=>=  NumberMaxEvents=1  SampleTime=Ts
  RTE Relational Operator3 : rteventslib/Math Operations/RTE Relational Operator  RelationalOperator=<=  NumberMaxEvents=1  SampleTime=Ts
  1 : Outport
  2 : Outport  Port=2
  3 : Outport  Port=3
  4 : Outport  Port=4
  wires:
  RTE Logical Operator/1 -> 3/1
  RTE Logical Operator1/1 -> 2/1
  RTE Relational Operator3/1 -> 4/1, RTE Logical Operator1/1
  RTE Relational Operator2/1 -> 1/1, RTE Logical Operator/1
  c-/1 -> RTE Relational Operator3/2
  c+/1 -> RTE Relational Operator2/2
  in/1 -> RTE Relational Operator2/1, RTE Relational Operator3/1

== system HVDC_VSC_1CPUcore_dcpl/SM_WSCC1_HVDCStation1/VSC Controller (Station 1)/3-level firing pulse unit for TSB/Subsystem6 ==
  in : Inport
  c+ : Inport  Port=2
  c- : Inport  Port=3
  RTE Logical Operator : rteventslib/Math Operations/RTE Logical Operator  LogicalOperator=NOT  NbrInput=1  NbrMaxEvents=1
  RTE Logical Operator1 : rteventslib/Math Operations/RTE Logical Operator  LogicalOperator=NOT  NbrInput=1  NbrMaxEvents=1
  RTE Relational Operator2 : rteventslib/Math Operations/RTE Relational Operator  RelationalOperator=>=  NumberMaxEvents=1  SampleTime=Ts
  RTE Relational Operator3 : rteventslib/Math Operations/RTE Relational Operator  RelationalOperator=<=  NumberMaxEvents=1  SampleTime=Ts
  1 : Outport
  2 : Outport  Port=2
  3 : Outport  Port=3
  4 : Outport  Port=4
  wires:
  RTE Logical Operator/1 -> 3/1
  RTE Logical Operator1/1 -> 2/1
  RTE Relational Operator3/1 -> 4/1, RTE Logical Operator1/1
  RTE Relational Operator2/1 -> 1/1, RTE Logical Operator/1
  c-/1 -> RTE Relational Operator3/2
  c+/1 -> RTE Relational Operator2/2
  in/1 -> RTE Relational Operator2/1, RTE Relational Operator3/1

== system HVDC_VSC_1CPUcore_dcpl/SM_WSCC1_HVDCStation1/VSC Controller (Station 1)/Discrete VSC Controller (Station 1)/Clark Transformations ==
  note: 0: Y-Y
      | 1: Y-D1
      | 2: Y-D11
  note: Clark's Transformations
  "U_abc " : Inport
  "I_abc " : Inport  Port=2
  "Uf_abc " : Inport  Port=3
  "Iv_abc " : Inport  Port=4
  "CLARK " : Subsystem  AncestorBlock=lib_mesures/CLARK
  "CLARK  " : Subsystem  AncestorBlock=lib_mesures/CLARK
  CLARK_YD : Subsystem
  "CLARK_YD " : Subsystem
  Constant2 : Constant  Value=Tr_connection
  Selector{,1..3} (4 alike) : Selector  InputPortWidth=3  Indices=[1 2]
  U_AB : Outport
  I_AB : Outport  Port=2
  Uf_AB : Outport  Port=3
  Iv_AB : Outport  Port=4
  wires:
  Constant2/1 -> "CLARK_YD "/2(Tr_conx), CLARK_YD/2(Tr_conx)
  "U_abc "/1 -> CLARK_YD/1(abc)
  "I_abc "/1 -> "CLARK_YD "/1(abc)
  "Uf_abc "/1 -> "CLARK "/1(abc)
  "Iv_abc "/1 -> "CLARK  "/1(abc)
  CLARK_YD/1(AB0) -> Selector/1
  "CLARK "/1(AB0) -> Selector2/1
  "CLARK  "/1(AB0) -> Selector3/1
  "CLARK_YD "/1(AB0) -> Selector1/1
  Selector/1 -> U_AB/1
  Selector1/1 -> I_AB/1
  Selector2/1 -> Uf_AB/1
  Selector3/1 -> Iv_AB/1
